simulink model "Regelung_mit_Beobachter_linear"  (R2021b)
settings: Solver=FixedStepAuto  StartTime=0.0  StopTime=25  FixedStep=1/1e4  RelTol=1e-3
undefined symbols (not defined in the file): A, B, C, L_LMI, start_deg, y_ref
settings Model: Creator=basti  LastModifiedBy=Aaron

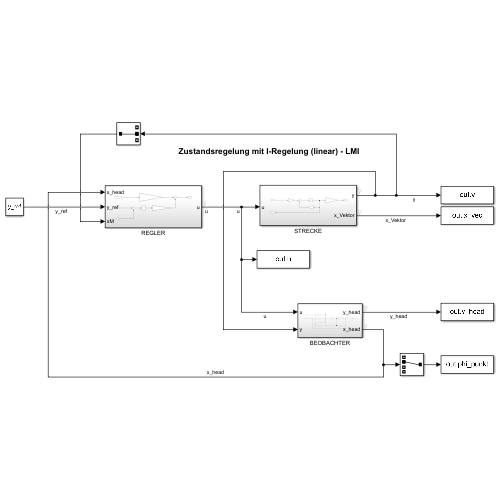
[thumbnail: Simulink's stored preview of the top-level diagram]
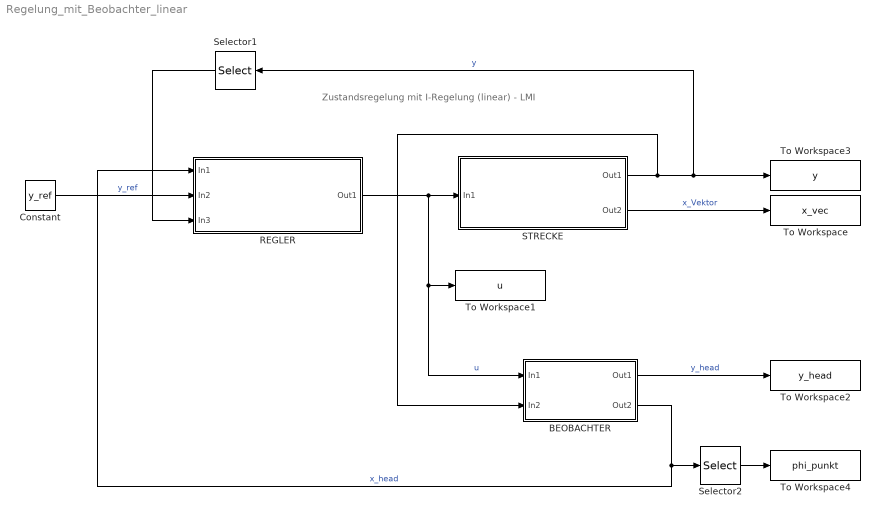
== system Regelung_mit_Beobachter_linear ==
  note: Zustandsregelung mit I-Regelung (linear) - LMI
  BEOBACHTER : Subsystem
  Constant : Constant  Value=y_ref
  REGLER : Subsystem
  STRECKE : Subsystem
  Selector1 : Selector  InputPortWidth=3  IndexOptions=Index vector (dialog)  Indices=2  OutputSizes=1
  Selector2 : Selector  InputPortWidth=4  IndexOptions=Index vector (dialog)  Indices=2  OutputSizes=1
  To Workspace : ToWorkspace  VariableName=x_vec  SaveFormat=Timeseries  SampleTime=-1
  To Workspace1 : ToWorkspace  VariableName=u  SaveFormat=Timeseries  SampleTime=-1
  To Workspace2 : ToWorkspace  VariableName=y_head  SaveFormat=Timeseries  SampleTime=-1
  To Workspace3 : ToWorkspace  VariableName=y  SaveFormat=Timeseries  SampleTime=-1
  To Workspace4 : ToWorkspace  VariableName=phi_punkt  SaveFormat=Timeseries  SampleTime=-1
  wires:
  STRECKE/1(Out1) -> BEOBACHTER/2(In2), Selector1/1, To Workspace3/1  "y"
  Constant/1 -> REGLER/2(In2)  "y_ref"
  REGLER/1(Out1) -> STRECKE/1(In1), BEOBACHTER/1(In1), To Workspace1/1  "u"
  STRECKE/2(Out2) -> To Workspace/1  "x_Vektor"
  BEOBACHTER/1(Out1) -> To Workspace2/1  "y_head"
  BEOBACHTER/2(Out2) -> Selector2/1, REGLER/1(In1)  "x_head"
  Selector1/1 -> REGLER/3(In3)
  Selector2/1 -> To Workspace4/1

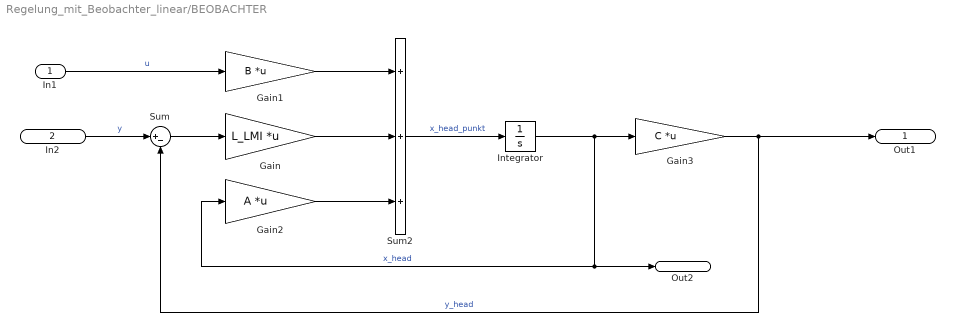
== system Regelung_mit_Beobachter_linear/BEOBACHTER ==
  In1 : Inport
  In2 : Inport  Port=2
  Gain : Gain  Gain=L_LMI  Multiplication=Matrix(K*u) (u vector)
  Gain1 : Gain  Gain=B  Multiplication=Matrix(K*u) (u vector)
  Gain2 : Gain  Gain=A  Multiplication=Matrix(K*u) (u vector)
  Gain3 : Gain  Gain=C  Multiplication=Matrix(K*u) (u vector)
  Integrator : Integrator
  Sum : Sum  Inputs=|+-
  Sum2 : Sum  Inputs=+++
  Out1 : Outport
  Out2 : Outport  Port=2
  wires:
  In1/1 -> Gain1/1  "u"
  Integrator/1 -> Out2/1, Gain2/1, Gain3/1  "x_head"
  Sum2/1 -> Integrator/1  "x_head_punkt"
  Gain1/1 -> Sum2/1
  Gain2/1 -> Sum2/3
  Gain/1 -> Sum2/2
  Gain3/1 -> Sum/2, Out1/1  "y_head"
  In2/1 -> Sum/1  "y"
  Sum/1 -> Gain/1

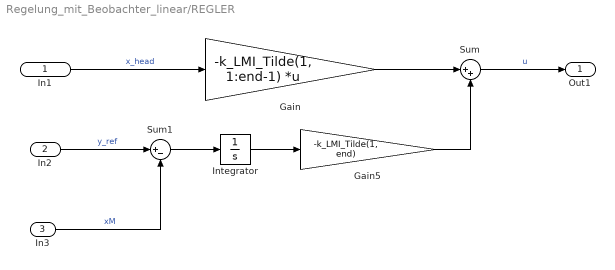
== system Regelung_mit_Beobachter_linear/REGLER ==
  In1 : Inport
  In2 : Inport  Port=2
  In3 : Inport  Port=3
  Gain : Gain  Gain=-k_LMI_Tilde(1, 1:end-1)  Multiplication=Matrix(K*u) (u vector)
  Gain5 : Gain  Gain=-k_LMI_Tilde(1, end)
  Integrator : Integrator
  Sum : Sum  Inputs=|++
  Sum1 : Sum  Inputs=|+-
  Out1 : Outport
  wires:
  Gain/1 -> Sum/1
  In1/1 -> Gain/1  "x_head"
  Sum/1 -> Out1/1  "u"
  In2/1 -> Sum1/1  "y_ref"
  In3/1 -> Sum1/2  "xM"
  Integrator/1 -> Gain5/1
  Sum1/1 -> Integrator/1
  Gain5/1 -> Sum/2

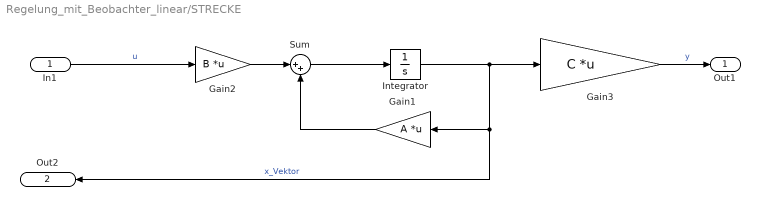
== system Regelung_mit_Beobachter_linear/STRECKE ==
  In1 : Inport
  Gain1 : Gain  Gain=A  Multiplication=Matrix(K*u) (u vector)
  Gain2 : Gain  Gain=B  Multiplication=Matrix(K*u) (u vector)
  Gain3 : Gain  Gain=C  Multiplication=Matrix(K*u) (u vector)
  Integrator : Integrator  InitialCondition=[(start_deg*pi)/180 0 0 0]
  Sum : Sum  Inputs=|++
  Out1 : Outport
  Out2 : Outport  Port=2
  wires:
  Gain1/1 -> Sum/2
  Gain3/1 -> Out1/1  "y"
  Sum/1 -> Integrator/1
  Integrator/1 -> Out2/1, Gain1/1, Gain3/1  "x_Vektor"
  Gain2/1 -> Sum/1
  In1/1 -> Gain2/1  "u"
